simulink model "SL_FT_a"  (R2019b)
settings: Solver=FixedStepDiscrete  StartTime=0.0  StopTime=6000  FixedStep=1  RelTol=1e-3  EnableMultiTasking=on
settings Model: SnapshotBufferSize=100  SnapshotInterval=1  Creator=dell  LastModifiedBy=DELL-PC
settings SolverCC: AutoInsertRateTranBlk=on
settings DataIOCC: LimitDataPoints=on  ReturnWorkspaceOutputs=off
settings OptimizationCC: LifeSpan=inf
settings DebuggingCC: AllowSymbolicDim=off  SFUnexpectedBacktrackingDiag=warning  SFNoUnconditionalDefaultTransitionDiag=warning  SFExecutionAtInitializationDiag=none  ArithmeticOperatorsInVariantConditions=warning
settings SFSimCC: SimUseLocalCustomCode=off  CustomCodeUndefinedFunction=UseInterfaceOnly
settings RTWCC: RTWUseLocalCustomCode=off
settings CodeAppCC: StateflowObjectComments=on
settings GRTTargetCC: TargetLangStandard=C89/C90 (ANSI)
settings ConfigComp: CovMetricSettings=dw  CovHtmlReporting=on  CovSaveCumulativeToWorkspaceVar=on  CovSaveSingleToWorkspaceVar=on  CovShowResultsExplorer=off  CovExternalEMLEnable=off

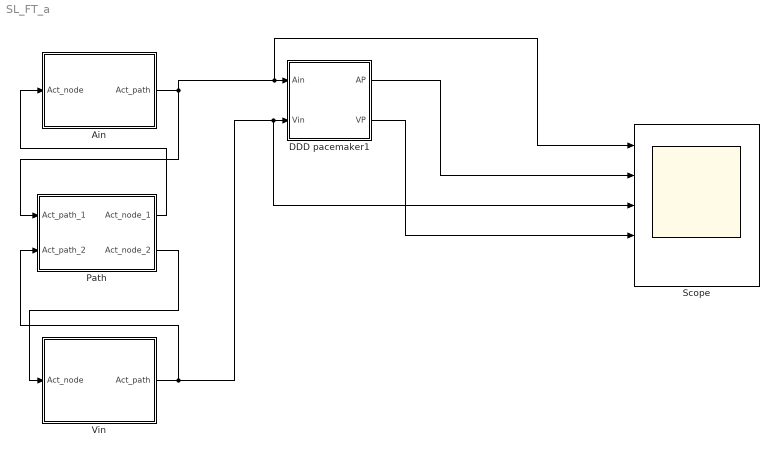
== system SL_FT_a ==
  Ain : Subsystem  AncestorBlock=model_library/Node
  DDD pacemaker1 : Subsystem
  Path : Subsystem  AncestorBlock=model_library/Path
  Scope : Scope  NumInputPorts=5
  "Vin " : Subsystem  AncestorBlock=model_library/Node
  wires:
  DDD pacemaker1/1(AP) -> Scope/2
  DDD pacemaker1/2(VP) -> Scope/4
  Ain/1(Act_path) -> Path/1(Act_path_1), DDD pacemaker1/1(Ain), Scope/1
  Path/2(Act_node_2) -> "Vin "/1(Act_node)
  "Vin "/1(Act_path) -> DDD pacemaker1/2(Vin), Scope/3, Path/2(Act_path_2)
  Path/1(Act_node_1) -> Ain/1(Act_node)

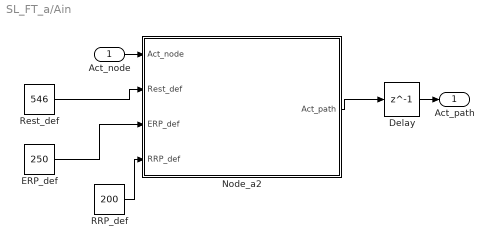
== system SL_FT_a/Ain ==
  Act_node : Inport
  Delay : Delay  DelayLength=1  InitialCondition=0
  ERP_def : Constant  Value=250  OutDataTypeStr=uint16
  Node_a2 : Stateflow chart  TreatAsAtomicUnit=on
  RRP_def : Constant  Value=200  OutDataTypeStr=uint16
  Rest_def : Constant  Value=546  OutDataTypeStr=uint16
  Act_path : Outport  VectorParamsAs1DForOutWhenUnconnected=off
  wires:
  RRP_def/1 -> Node_a2/4(RRP_def)
  Delay/1 -> Act_path/1
  ERP_def/1 -> Node_a2/3(ERP_def)
  Rest_def/1 -> Node_a2/2(Rest_def)
  Act_node/1 -> Node_a2/1(Act_node)
  Node_a2/1(Act_path) -> Delay/1

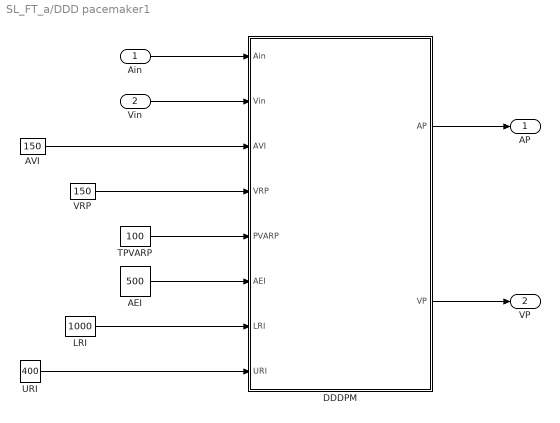
== system SL_FT_a/DDD pacemaker1 ==
  Ain : Inport
  Vin : Inport  Port=2
  AEI : Constant  Value=500
  AVI : Constant  Value=150  OutDataTypeStr=uint16
  DDDPM : Stateflow chart  TreatAsAtomicUnit=on
  LRI : Constant  Value=1000  OutDataTypeStr=uint16
  TPVARP : Constant  Value=100  OutDataTypeStr=uint16
  URI : Constant  Value=400  OutDataTypeStr=uint16
  VRP : Constant  Value=150  OutDataTypeStr=uint16
  AP : Outport
  VP : Outport  Port=2
  wires:
  DDDPM/2(VP) -> VP/1
  DDDPM/1(AP) -> AP/1
  Vin/1 -> DDDPM/2(Vin)
  Ain/1 -> DDDPM/1(Ain)
  AVI/1 -> DDDPM/3(AVI)
  VRP/1 -> DDDPM/4(VRP)
  TPVARP/1 -> DDDPM/5(PVARP)
  URI/1 -> DDDPM/8(URI)
  LRI/1 -> DDDPM/7(LRI)
  AEI/1 -> DDDPM/6(AEI)

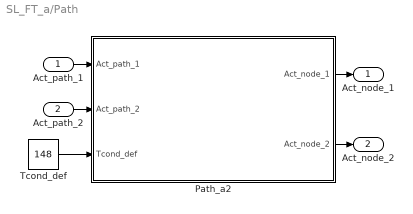
== system SL_FT_a/Path ==
  Act_path_1 : Inport
  Act_path_2 : Inport  Port=2
  Path_a2 : Stateflow chart  TreatAsAtomicUnit=on
  Tcond_def : Constant  Value=148  OutDataTypeStr=uint16
  Act_node_1 : Outport  VectorParamsAs1DForOutWhenUnconnected=off
  Act_node_2 : Outport  Port=2  VectorParamsAs1DForOutWhenUnconnected=off
  wires:
  Tcond_def/1 -> Path_a2/3(Tcond_def)
  Path_a2/2(Act_node_2) -> Act_node_2/1
  Act_path_1/1 -> Path_a2/1(Act_path_1)
  Act_path_2/1 -> Path_a2/2(Act_path_2)
  Path_a2/1(Act_node_1) -> Act_node_1/1

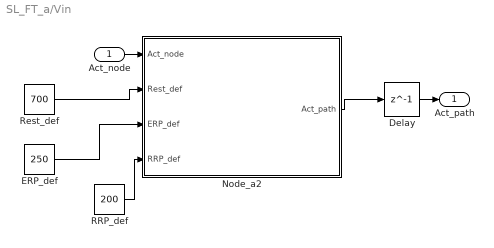
== system SL_FT_a/Vin  ==
  Act_node : Inport
  Delay : Delay  DelayLength=1  InitialCondition=0
  ERP_def : Constant  Value=250  OutDataTypeStr=uint16
  Node_a2 : Stateflow chart  TreatAsAtomicUnit=on
  RRP_def : Constant  Value=200  OutDataTypeStr=uint16
  Rest_def : Constant  Value=700  OutDataTypeStr=uint16
  Act_path : Outport  VectorParamsAs1DForOutWhenUnconnected=off
  wires:
  RRP_def/1 -> Node_a2/4(RRP_def)
  Delay/1 -> Act_path/1
  ERP_def/1 -> Node_a2/3(ERP_def)
  Rest_def/1 -> Node_a2/2(Rest_def)
  Act_node/1 -> Node_a2/1(Act_node)
  Node_a2/1(Act_path) -> Delay/1

== stateflow chart SL_FT_a/Vin /Node_a2 ==
  state node
    settings: description=|
        | temp can be thought of a sub-mode of ERP, which only exists to make sure that act_path is high for one period.
        | 
        | In ERP, if Act_node is received, then it is ignored through that self-transition.
        | 
        | Note this doesn't model variations in cycle length because everytime it is stimulated in RRP, ERP_cur is set to ERP_def again.
    state Rest
    state RRP
    state ERP
    state temp
    (default) -> Rest : {Rest_cur=Rest_def;}
    Rest -> temp [order 3] : [Act_node==false && Rest_cur<=uint16(0)]/{Act_path=true;uptime= uint16(0);ERP_cur=ERP_def;}
    Rest -> temp [order 1] : [Act_node==true]/{Act_path=true;uptime= uint16(0);ERP_cur=ERP_def;}
    Rest -> Rest [order 2] : [Act_node==false && Rest_cur>uint16(0)]/{Rest_cur = Rest_cur - uint16(1);}
    RRP -> Rest [order 1] : [RRP_cur<=0]/{Rest_cur=Rest_def;}
    RRP -> RRP [order 2] : [Act_node==false && RRP_cur>0]/{RRP_cur=RRP_cur-uint16(1);}
    RRP -> temp [order 3] : [Act_node==true]/{Act_path=true;uptime= uint16(0);ERP_cur=ERP_def;}
    ERP -> RRP [order 1] : [ERP_cur<=uint16(0)]/{RRP_cur=RRP_def;}
    temp -> temp [order 1] : [uptime<uint16(1)]/{uptime = uptime + uint16(1);ERP_cur =ERP_cur - uint16(1);}
    temp -> ERP [order 2] : [uptime>=uint16(1)]/{Act_path=false;}
    ERP -> ERP [order 3] : [Act_node==true]
    ERP -> ERP [order 2] : {ERP_cur = ERP_cur - uint16(1);}
  data: Act_node input boolean; Act_path output boolean; Rest_cur local uint16; ERP_cur local uint16; Rest_def input uint16; ERP_def input uint16; uptime local uint16; RRP_cur local uint16; RRP_def input uint16

== stateflow chart SL_FT_a/DDD pacemaker1/DDDPM ==
  settings: updateMethod=DISCRETE  sampleTime=1
  state DDDPM
    state AVI [parallel]
      settings: executionOrder=3
      state ActiveAVI
      state CAVI
      state IdleAVI
      (default) -> IdleAVI : {VP=false,VP1=false;}
      ActiveAVI -> ActiveAVI [order 3] : [tmpAVI>0]/{tmpAVI=tmpAVI-1;}
      IdleAVI -> ActiveAVI : [AS==true || AP1==true]/
          | {tmpAVI=AVI;}
      ActiveAVI -> CAVI [order 1] : [tmpAVI<=0&&enterURI==true]/
          | {VP=true, VP1=true;}
      ActiveAVI -> IdleAVI [order 2] : [VS==true || VP1==true]
      CAVI -> IdleAVI : {VP=false,VP1=false;}
    state URI [parallel]
      settings: executionOrder=1
      state IdleURI
      state ActiveURI
      (default) -> IdleURI : {enterURI=true;}
      IdleURI -> ActiveURI : [VP1==true || VS==true]/
          | {tmpURI=URI, enterURI=false;}
      ActiveURI -> IdleURI [order 3] : [tmpURI<=0]/{enterURI=true;}
      ActiveURI -> ActiveURI [order 2] : [tmpURI>0]/{tmpURI = tmpURI - 1;}
      ActiveURI -> ActiveURI [order 1] : [VS==true || VP1==true]/
          | {tmpURI=URI, enterURI=false;}
    state PVARP [parallel]
      settings: executionOrder=5
      state AinPVARP
      state IdlePVARP
      state ActivePVARP
      state PVARPAR
      IdlePVARP -> AinPVARP [order 1] : [Ain==true]/{AS=true}
      AinPVARP -> IdlePVARP : {AS=false;}
      (default) -> IdlePVARP : {AS=false;}
      IdlePVARP -> ActivePVARP [order 2] : [VS==true || VP1==true]/{tmpPVARP=PVARP;}
      ActivePVARP -> IdlePVARP [order 3] : [tmpPVARP<=0]
      ActivePVARP -> ActivePVARP [order 2] : [tmpPVARP>0]/
          | {tmpPVARP = tmpPVARP - 1;}
      PVARPAR -> ActivePVARP : {AR=false,tmpPVARP = tmpPVARP - 1;}
      ActivePVARP -> PVARPAR [order 1] : [Ain==true]/{AR=true;}
    state LRI [parallel]
      settings: executionOrder=2
      state IdleLRI
      state LRIVP
      state ActiveLRI
      IdleLRI -> IdleLRI [order 1] : [VS==true||VP1==true]/
          | {tmpLRI=LRI;}
      (default) -> IdleLRI : {tmpLRI = LRI,APLRI=2,AP=false,AP1=false;}
      IdleLRI -> IdleLRI [order 3] : [tmpLRI>AVI]/
          | {tmpLRI = tmpLRI-1;}
      LRIVP -> IdleLRI : /{VP=false, VP1=false, tmpLRI=LRI;}
      IdleLRI -> ActiveLRI [order 4] : [tmpLRI<=AVI]/
          | {AP=true,APLRI=1,AP1=true,tmpLRI=tmpLRI-1;}
      IdleLRI -> ActiveLRI [order 2] : [AS==true]/{tmpLRI=tmpLRI-1;}
      ActiveLRI -> IdleLRI [order 2] : [VS==true || VP1==true]/{tmpLRI=LRI;}
      ActiveLRI -> LRIVP [order 4] : [tmpLRI<=0]/
          | {VP=true,VP1=true;}
      ActiveLRI -> ActiveLRI [order 3] : [tmpLRI>0]
          | /{tmpLRI=tmpLRI-1;}
      ActiveLRI -> ActiveLRI [order 1] : [APLRI==1]/
          | {APLRI=APLRI+1,AP=false,AP1=false,
          | tmpLRI=tmpLRI-1;}
    state VRP [parallel]
      settings: executionOrder=4
      state VRPVS
      state IdleVRP
      state ActiveVRP
      IdleVRP -> VRPVS [order 1] : [Vin==true]/{VS=true}
      VRPVS -> ActiveVRP : {tmpVRP=VRP,VS=false;}
      (default) -> IdleVRP : {VS=false}
      IdleVRP -> ActiveVRP [order 2] : [VP1==true]/{tmpVRP=VRP;}
      ActiveVRP -> ActiveVRP [order 1] : [tmpVRP>0]/{tmpVRP= tmpVRP - 1;}
      ActiveVRP -> IdleVRP [order 2] : [tmpVRP<=0]
  (default) -> DDDPM : {VS=false, VP1=false, VP=false, AS=false,AR=false,AP1=false,  APLRI=2,  AP=false,  enterURI=true, tmpVRP=VRP, tmpPVARP = PVARP, tmpAVI= AVI, tmpLRI = LRI, tmpURI = URI;}
  data: Ain input; VS local; Vin input; AP output; VP output; tmpVRP local; AS local; tmpPVARP local; tmpAVI local; enterURI local; tmpLRI local; tmpURI local; APLRI local; VP1 local; AP1 local; AR local; AVI input uint16; VRP input uint16 =150; PVARP input uint16; AEI input; LRI input uint16; URI input uint16; APLRI1 local

== stateflow chart SL_FT_a/Ain/Node_a2 ==
  state node
    settings: description=|
        | temp can be thought of a sub-mode of ERP, which only exists to make sure that act_path is high for one period.
        | 
        | In ERP, if Act_node is received, then it is ignored through that self-transition.
        | 
        | Note this doesn't model variations in cycle length because everytime it is stimulated in RRP, ERP_cur is set to ERP_def again.
    state Rest
    state RRP
    state ERP
    state temp
    (default) -> Rest : {Rest_cur=Rest_def;}
    Rest -> temp [order 3] : [Act_node==false && Rest_cur<=uint16(0)]/{Act_path=true;uptime= uint16(0);ERP_cur=ERP_def;}
    Rest -> temp [order 1] : [Act_node==true]/{Act_path=true;uptime= uint16(0);ERP_cur=ERP_def;}
    Rest -> Rest [order 2] : [Act_node==false && Rest_cur>uint16(0)]/{Rest_cur = Rest_cur - uint16(1);}
    RRP -> Rest [order 1] : [RRP_cur<=0]/{Rest_cur=Rest_def;}
    RRP -> RRP [order 2] : [Act_node==false && RRP_cur>0]/{RRP_cur=RRP_cur-uint16(1);}
    RRP -> temp [order 3] : [Act_node==true]/{Act_path=true;uptime= uint16(0);ERP_cur=ERP_def;}
    ERP -> RRP [order 1] : [ERP_cur<=uint16(0)]/{RRP_cur=RRP_def;}
    temp -> temp [order 1] : [uptime<uint16(1)]/{uptime = uptime + uint16(1);ERP_cur =ERP_cur - uint16(1);}
    temp -> ERP [order 2] : [uptime>=uint16(1)]/{Act_path=false;}
    ERP -> ERP [order 3] : [Act_node==true]
    ERP -> ERP [order 2] : {ERP_cur = ERP_cur - uint16(1);}
  data: Act_node input boolean; Act_path output boolean; Rest_cur local uint16; ERP_cur local uint16; Rest_def input uint16; ERP_def input uint16; uptime local uint16; RRP_cur local uint16; RRP_def input uint16

== stateflow chart SL_FT_a/Path/Path_a2 ==
  state path
    state Idle
    state Ante
    state Retro
    state Wait
    (default) -> Idle
    Idle -> Ante [order 1] : [Act_path_1==true]/{Tcond_cur=Tcond_def;}
    Idle -> Retro [order 2] : [Act_path_2==true]/{Tcond_cur=Tcond_def;}
    Wait -> Idle [order 1] : [uptime>0]/{Act_node_1=false;Act_node_2=false;}
    Ante -> Ante [order 3] : [Act_path_2==false && Tcond_cur>uint16(0)]/{Tcond_cur = Tcond_cur - uint16(1);}
    Retro -> Retro [order 3] : [Act_path_1==false && Tcond_cur>uint16(0)]/{Tcond_cur = Tcond_cur - uint16(1);}
    Ante -> Wait [order 2] : [Act_path_2==true]/{uptime=uint16(0);}
    Ante -> Wait [order 1] : [Act_path_2==false && Tcond_cur<=uint16(0)]/{Act_node_2=true;uptime=uint16(0);}
    Retro -> Wait [order 2] : [Act_path_1==true]/{uptime=uint16(0);}
    Retro -> Wait [order 1] : [Act_path_1==false && Tcond_cur<=uint16(0)]/{Act_node_1=true;uptime=uint16(0);}
    Wait -> Wait [order 2] : [uptime<=uint16(0)]/{uptime = uptime + uint16(1);}
  data: Act_path_1 input boolean; Act_path_2 input boolean; Act_node_1 output boolean; Act_node_2 output boolean; Tcond_cur local uint16; Tcond_def input uint16; uptime local uint16
